simulink model "Design"  (R2023b)
settings: Solver=VariableStepAuto  StartTime=0.0  StopTime=10.0  RelTol=1e-3
libraries: cstblocks x5
settings Model: Creator=PierluigiMeneses  LastModifiedBy=PierluigiMeneses

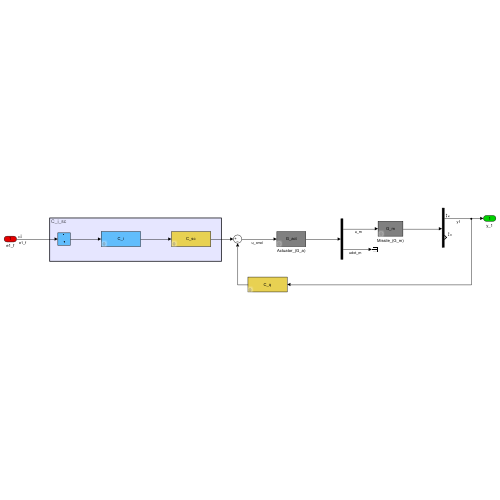
[thumbnail: Simulink's stored preview of the top-level diagram]
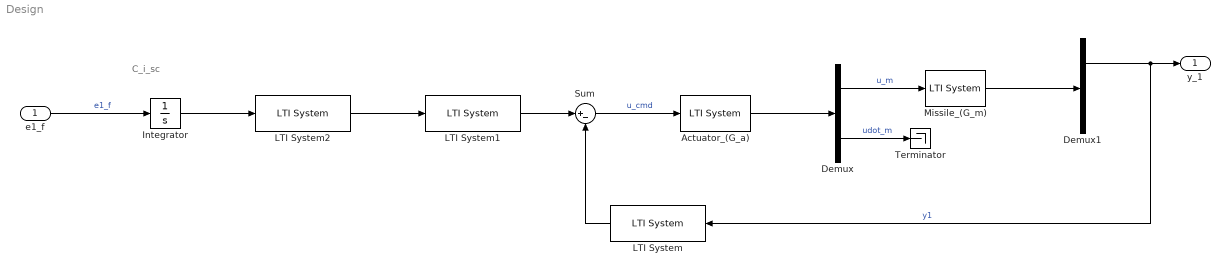
== system Design ==
  note: C_i_sc
  e1_f : Inport
  Actuator_(G_a) : cstblocks/LTI System  sys=G_act  IC=[]  PadeOrder=0
  Demux : Demux  Outputs=2
  Demux1 : Demux  Outputs=2
  Integrator : Integrator
  LTI System : cstblocks/LTI System  sys=C_q  IC=[]  PadeOrder=0
  LTI System1 : cstblocks/LTI System  sys=C_sc  IC=[]  PadeOrder=0
  LTI System2 : cstblocks/LTI System  sys=C_i  IC=[]  PadeOrder=0
  Missile_(G_m) : cstblocks/LTI System  sys=G_m  IC=[]  PadeOrder=0
  Sum : Sum  Inputs=|+-
  Terminator : Terminator
  y_1 : Outport
  wires:
  Sum/1 -> Actuator_(G_a)/1  "u_cmd"
  Demux1/1 -> LTI System/1, y_1/1  "y1"
  Integrator/1 -> LTI System2/1
  e1_f/1 -> Integrator/1  "e1_f"
  LTI System2/1 -> LTI System1/1
  Missile_(G_m)/1 -> Demux1/1
  Demux/2 -> Terminator/1  "udot_m"
  Actuator_(G_a)/1 -> Demux/1
  Demux/1 -> Missile_(G_m)/1  "u_m"
  LTI System/1 -> Sum/2
  LTI System1/1 -> Sum/1
